simulink model "simulated_lab2_1"  (Simulink 8.9)
settings: Solver=VariableStepAuto  StartTime=0.0  StopTime=10.0  RelTol=1e-3
undefined symbols (not defined in the file or in its folder): B, M
settings Model: Creator=c3204612  LastModifiedBy=Administrator
settings DataIOCC: LimitDataPoints=off  SaveFormat=Dataset  SignalLoggingSaveFormat=Dataset
settings DebuggingCC: UnderspecifiedInitializationDetection=Simplified  MergeDetectMultiDrivingBlocksExec=error  FcnCallInpInsideContextMsg=error  StateNameClashWarn=none  SFUnexpectedBacktrackingDiag=error  SFNoUnconditionalDefaultTransitionDiag=error
settings HardwareCC: ProdBitPerPointer=64  ProdBitPerSizeT=64  ProdBitPerPtrDiffT=64  ProdLargestAtomicFloat=Float  ProdIntDivRoundTo=Zero  ProdEndianess=LittleEndian  ProdWordSize=64  ProdHWDeviceType=Intel->x86-64 (Windows64)
settings ModelReferenceCC: PropagateSignalLabelsOutOfModel=on
settings GRTTargetCC: TargetLangStandard=C99 (ISO)  GeneratePreprocessorConditionals=Use local settings  CombineOutputUpdateFcns=on  GRTInterface=off
settings ConfigComp: CovMetricSettings=dwe  CovHtmlReporting=off  CovSaveCumulativeToWorkspaceVar=off  CovSaveSingleToWorkspaceVar=off  CovExternalEMLEnable=on

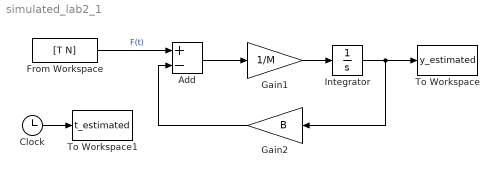
== system simulated_lab2_1 ==
  Add : Sum  Inputs=+-
  Clock : Clock
  From Workspace : FromWorkspace  VariableName=[T N]  SampleTime=0
  Gain1 : Gain  Gain=1/M
  Gain2 : Gain  Gain=B
  Integrator : Integrator
  To Workspace : ToWorkspace  VariableName=y_estimated  SampleTime=-1
  To Workspace1 : ToWorkspace  VariableName=t_estimated  SampleTime=-1
  wires:
  From Workspace/1 -> Add/1  "F(t)"
  Add/1 -> Gain1/1
  Gain1/1 -> Integrator/1
  Integrator/1 -> Gain2/1, To Workspace/1
  Gain2/1 -> Add/2
  Clock/1 -> To Workspace1/1
